simulink model "program_nova_torque_vectoring_001_2015b"  (R2016a)
settings: Solver=FixedStepAuto  StartTime=0.0  StopTime=10.0  RelTol=1e-3
PreLoadFcn:
  | dataCar
  | load_vars
  | readFuzzyFile
  | structAero
  | structEstimPar
  | structSensors
  | structSettings
PostLoadFcn:
  | , if any(exist('dsrtsu_mdlpostloadfcn', 'file') == [2, 3, 6]), try dsrtsu_mdlpostloadfcn('Execute', bdroot); catch fprintf('Error in PostLoadFcn (dsrtsu_mdlpostloadfcn) for model "%s":\n %s\n', bdroot, lasterr); end, end,
InitFcn:
  | dataCar
  | load_vars
  | readFuzzyFile
  | structAero
  | structEstimPar
  | structSensors
  | structSettings
StartFcn:
  | dataCar
  | load_vars
  | readFuzzyFile
  | structAero
  | structEstimPar
  | structSensors
  | structSettings
values from neighbouring files (symbols this model uses):
  Throttle2_offset = 500    [load_vars.m]
  Throttle_limits = [0.15, 0.90, 0.16, 0.92]    [load_vars.m]
libraries: rtican x42, hdlsllib x32, simulink x3, fuzblock x1
(part 10 of 11)

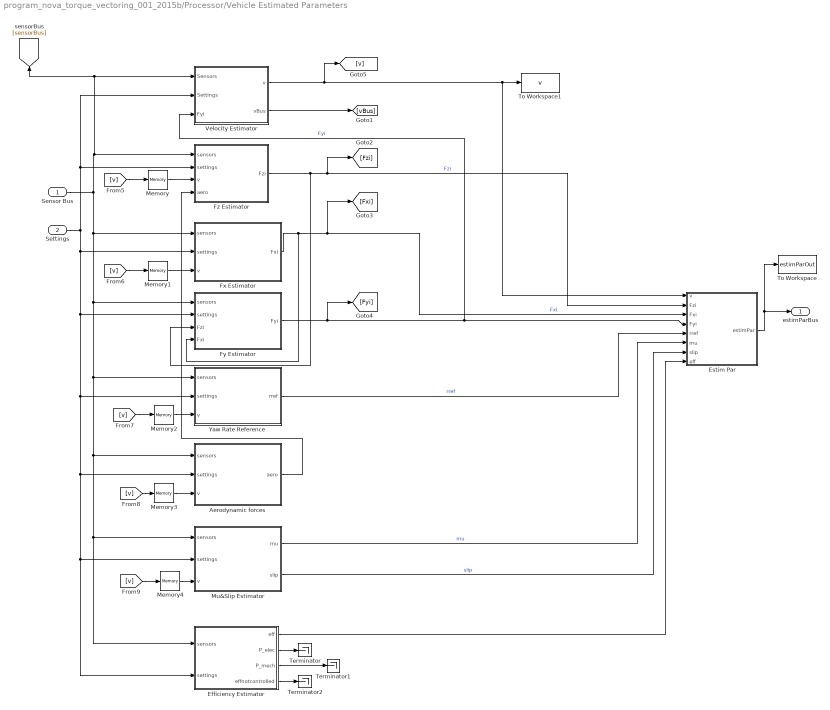
== system program_nova_torque_vectoring_001_2015b/Processor/Vehicle Estimated Parameters ==
  Sensor Bus : Inport
  Settings : Inport  Port=2
  Aerodynamic forces : MATLAB Function  TreatAsAtomicUnit=on
  Efficiency Estimator : MATLAB Function  TreatAsAtomicUnit=on
  Estim Par : MATLAB Function  TreatAsAtomicUnit=on
  "Fx Estimator " : MATLAB Function  TreatAsAtomicUnit=on
  "Fy Estimator " : MATLAB Function  TreatAsAtomicUnit=on
  "Fz Estimator " : MATLAB Function  TreatAsAtomicUnit=on
  Memory{,1..4} (5 alike) : Memory
  Mu&Slip Estimator : MATLAB Function  TreatAsAtomicUnit=on
  Terminator : Terminator
  Terminator1 : Terminator
  Terminator2 : Terminator
  To Workspace : ToWorkspace  VariableName=estimParOut  SaveFormat=Timeseries  SampleTime=-1
  To Workspace1 : ToWorkspace  VariableName=v  SaveFormat=Timeseries  SampleTime=-1
  Velocity Estimator : Subsystem
  Yaw Rate Reference : MATLAB Function  TreatAsAtomicUnit=on
  " estimParBus" : Outport
  wires:
  "Fx Estimator "/1(Fxi) -> Estim Par/3(Fxi), [Fxi], "Fy Estimator "/4(Fxi)  "Fxi"
  "Fz Estimator "/1(Fzi) -> "Fy Estimator "/3(Fzi), Estim Par/2(Fzi), [Fzi]  "Fzi"
  Yaw Rate Reference/1(rref) -> Estim Par/5(rref)  "rref"
  "Fy Estimator "/1(Fyi) -> Velocity Estimator/3(Fyi), Estim Par/4(Fyi), [Fyi]  "Fyi"
  Estim Par/1(estimPar) -> To Workspace/1, " estimParBus"/1
  Sensor Bus/1 -> "Fx Estimator "/1(sensors), Efficiency Estimator/1(sensors), Mu&Slip Estimator/1(sensors), Aerodynamic forces/1(sensors), Yaw Rate Reference/1(sensors), "Fy Estimator "/1(sensors), "Fz Estimator "/1(sensors), Velocity Estimator/1(Sensors), [sensorBus]
  Settings/1 -> Velocity Estimator/2(Settings), "Fz Estimator "/2(settings), Efficiency Estimator/2(settings), Mu&Slip Estimator/2(settings), Aerodynamic forces/2(settings), Yaw Rate Reference/2(settings), "Fy Estimator "/2(settings), "Fx Estimator "/2(settings)
  Velocity Estimator/1(v) -> [v], To Workspace1/1, Estim Par/1(v)
  Velocity Estimator/2(vBus) -> [vBus]
  Aerodynamic forces/1(aero) -> "Fz Estimator "/4(aero)
  Mu&Slip Estimator/1(mu) -> Estim Par/6(mu)  "mu"
  Mu&Slip Estimator/2(slip) -> Estim Par/7(slip)  "slip"
  [v] -> Memory/1
  [v] -> Memory1/1
  [v] -> Memory2/1
  [v] -> Memory3/1
  [v] -> Memory4/1
  Memory/1 -> "Fz Estimator "/3(v)
  Memory1/1 -> "Fx Estimator "/3(v)
  Memory2/1 -> Yaw Rate Reference/3(v)
  Memory3/1 -> Aerodynamic forces/3(v)
  Memory4/1 -> Mu&Slip Estimator/3(v)
  Efficiency Estimator/1(eff) -> Estim Par/8(eff)
  Efficiency Estimator/4(effnotcontrolled) -> Terminator2/1
  Efficiency Estimator/2(P_elec) -> Terminator/1
  Efficiency Estimator/3(P_mech) -> Terminator1/1

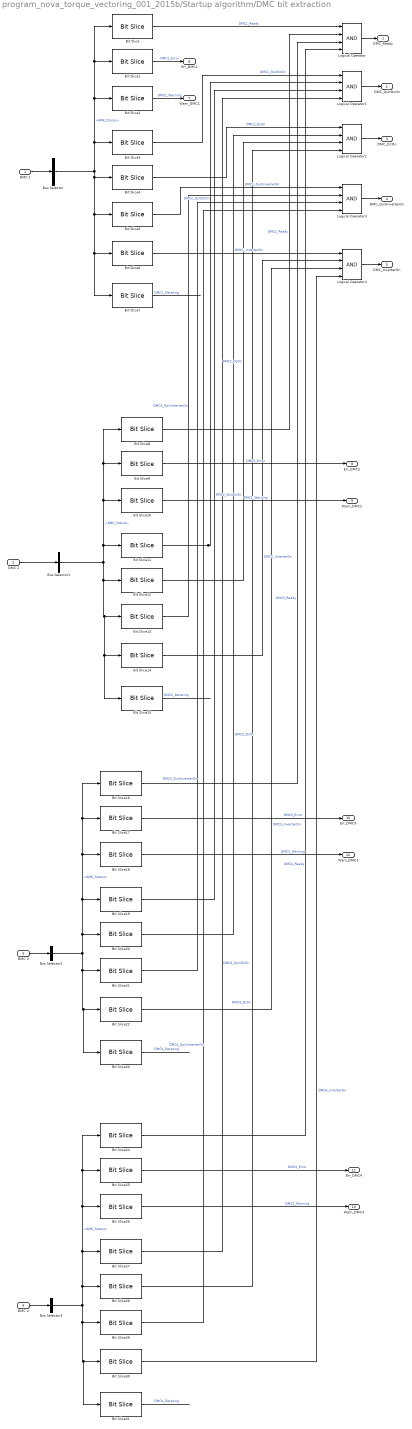
== system program_nova_torque_vectoring_001_2015b/Startup algorithm/DMC bit extraction ==
  DMC 1 : Inport
  DMC 2 : Inport  Port=2
  DMC 3 : Inport  Port=3
  DMC 4 : Inport  Port=4
  Bit Slice{,8,16,24} (4 alike) : hdlsllib/HDL Operations/Bit Slice  lidx=8  ridx=8
  Bit Slice{1,9,17,25} (4 alike) : hdlsllib/HDL Operations/Bit Slice  lidx=9  ridx=9
  Bit Slice{2,10,18,26} (4 alike) : hdlsllib/HDL Operations/Bit Slice  lidx=10  ridx=10
  Bit Slice{3,11,19,27} (4 alike) : hdlsllib/HDL Operations/Bit Slice  lidx=11  ridx=11
  Bit Slice{4,12,20,28} (4 alike) : hdlsllib/HDL Operations/Bit Slice  lidx=12  ridx=12
  Bit Slice{5,13,21,29} (4 alike) : hdlsllib/HDL Operations/Bit Slice  lidx=13  ridx=13
  Bit Slice{6,14,22,30} (4 alike) : hdlsllib/HDL Operations/Bit Slice  lidx=14  ridx=14
  Bit Slice{7,15,23,31} (4 alike) : hdlsllib/HDL Operations/Bit Slice  lidx=15  ridx=15
  Bus Selector{,1..3} (4 alike) : BusSelector  OutputSignals=AMK_Status
  Logical Operator{,1..4} (5 alike) : Logic  Inputs=4  AllPortsSameDT=off  OutDataTypeStr=boolean
  DMC_Ready : Outport
  DMC_QuitDcOn : Outport  Port=2
  DMC_DcOn : Outport  Port=3
  DMC_QuitInverterOn : Outport  Port=4
  DMC_InverterOn : Outport  Port=5
  Err_DMC1 : Outport  Port=6
  Warn_DMC1 : Outport  Port=7
  Err_DMC2 : Outport  Port=8
  Warn_DMC2 : Outport  Port=9
  Err_DMC3 : Outport  Port=10
  Err_DMC4 : Outport  Port=11
  Warn_DMC3 : Outport  Port=12
  Warn_DMC4 : Outport  Port=13
  wires:
  DMC 4/1 -> Bus Selector3/1
  DMC 3/1 -> Bus Selector2/1
  DMC 1/1 -> Bus Selector/1
  DMC 2/1 -> Bus Selector1/1
  Bus Selector/1 -> Bit Slice7/1, Bit Slice6/1, Bit Slice5/1, Bit Slice4/1, Bit Slice/1, Bit Slice1/1, Bit Slice2/1, Bit Slice3/1  "<AMK_Status>"
  Bit Slice/1 -> Logical Operator/1  "DMC1_Ready"
  Bit Slice1/1 -> Err_DMC1/1  "DMC1_Error"
  Bit Slice2/1 -> Warn_DMC1/1  "DMC1_Warning"
  Bit Slice3/1 -> Logical Operator1/1  "DMC1_QuitDcOn"
  Bit Slice4/1 -> Logical Operator2/1  "DMC1_DcOn"
  Bit Slice5/1 -> Logical Operator3/1  "DMC1_QuitInverterOn"
  Bit Slice6/1 -> Logical Operator4/1  "DMC1_InverterOn"
  Bit Slice7/1 -> ?  "DMC1_Derating"
  Bus Selector1/1 -> Bit Slice15/1, Bit Slice14/1, Bit Slice13/1, Bit Slice12/1, Bit Slice8/1, Bit Slice9/1, Bit Slice10/1, Bit Slice11/1  "<AMK_Status>"
  Bit Slice8/1 -> Logical Operator/2  "DMC2_Ready"
  Bit Slice9/1 -> Err_DMC2/1  "DMC2_Error"
  Bit Slice10/1 -> Warn_DMC2/1  "DMC2_Warning"
  Bit Slice11/1 -> Logical Operator1/2  "DMC2_QuitDcOn"
  Bit Slice12/1 -> Logical Operator2/3  "DMC2_DcOn"
  Bit Slice13/1 -> Logical Operator3/2  "DMC2_QuitInverterOn"
  Bit Slice14/1 -> Logical Operator4/2  "DMC2_InverterOn"
  Bit Slice15/1 -> ?  "DMC2_Derating"
  Bus Selector2/1 -> Bit Slice16/1, Bit Slice17/1, Bit Slice18/1, Bit Slice19/1, Bit Slice20/1, Bit Slice23/1, Bit Slice22/1, Bit Slice21/1  "<AMK_Status>"
  Bit Slice16/1 -> Logical Operator/3  "DMC3_Ready"
  Bit Slice17/1 -> Err_DMC3/1  "DMC3_Error"
  Bit Slice18/1 -> Warn_DMC3/1  "DMC3_Warning"
  Bit Slice19/1 -> Logical Operator1/3  "DMC3_QuitDcOn"
  Bit Slice20/1 -> Logical Operator2/2  "DMC3_DcOn"
  Bit Slice21/1 -> Logical Operator3/3  "DMC3_QuitInverterOn"
  Bit Slice22/1 -> Logical Operator4/3  "DMC3_InverterOn"
  Bit Slice23/1 -> ?  "DMC3_Derating"
  Bus Selector3/1 -> Bit Slice24/1, Bit Slice25/1, Bit Slice26/1, Bit Slice27/1, Bit Slice28/1, Bit Slice31/1, Bit Slice30/1, Bit Slice29/1  "<AMK_Status>"
  Bit Slice24/1 -> Logical Operator/4  "DMC4_Ready"
  Bit Slice25/1 -> Err_DMC4/1  "DMC4_Error"
  Bit Slice26/1 -> Warn_DMC4/1  "DMC4_Warning"
  Bit Slice27/1 -> Logical Operator1/4  "DMC4_QuitDcOn"
  Bit Slice28/1 -> Logical Operator2/4  "DMC4_DcOn"
  Bit Slice29/1 -> Logical Operator3/4  "DMC4_QuitInverterOn"
  Bit Slice30/1 -> Logical Operator4/4  "DMC4_InverterOn"
  Bit Slice31/1 -> ?  "DMC4_Derating"
  Logical Operator/1 -> DMC_Ready/1
  Logical Operator1/1 -> DMC_QuitDcOn/1
  Logical Operator2/1 -> DMC_DcOn/1
  Logical Operator3/1 -> DMC_QuitInverterOn/1
  Logical Operator4/1 -> DMC_InverterOn/1

== system program_nova_torque_vectoring_001_2015b/Startup algorithm/Merge_Controlword ==
  Control_in : Inport
  DcOn : Inport  Port=2
  Enable : Inport  Port=3
  InverterOn : Inport  Port=4
  ErrorReset : Inport  Port=5
  Bus Creator : BusCreator  Inputs=4
  If CTRL = Null : MATLAB Function  TreatAsAtomicUnit=on
  Control : Outport
  wires:
  Enable/1 -> If CTRL = Null/3(En_in)
  InverterOn/1 -> If CTRL = Null/4(Inv_in)
  DcOn/1 -> If CTRL = Null/2(Dc_in)
  Control_in/1 -> If CTRL = Null/1(Ctrl_in)
  If CTRL = Null/1(DcOn) -> Bus Creator/1
  If CTRL = Null/2(Enable) -> Bus Creator/2
  If CTRL = Null/3(InverterOn) -> Bus Creator/3
  Bus Creator/1 -> Control/1  "Controlbits"
  ErrorReset/1 -> Bus Creator/4  "ErrorReset"

== system program_nova_torque_vectoring_001_2015b/Processor/Control Systems/Distributor ==
  sensors : Inport
  settings : Inport  Port=2
  estimPar : Inport  Port=3
  Mz : Inport  Port=4
  MATLAB Function : MATLAB Function  TreatAsAtomicUnit=on
  MdesFdesFxmaxFx : Scope  NumInputPorts=4
  Mux : Mux
  To Workspace : ToWorkspace  VariableName=Fdes  SaveFormat=Timeseries  SampleTime=-1
  To Workspace1 : ToWorkspace  VariableName=Fxmax  SaveFormat=Timeseries  SampleTime=-1
  To Workspace2 : ToWorkspace  VariableName=MdesFdesFxmaxFx  SaveFormat=Timeseries  SampleTime=-1
  To Workspace4 : ToWorkspace  VariableName=Fx  SaveFormat=Timeseries  SampleTime=-1
  Torque/Brake analyzer : Subsystem
  torqueDistribution : Outport
  slipSet : Outport  Port=2
  wires:
  MATLAB Function/1(torqueDistribution) -> torqueDistribution/1
  sensors/1 -> Torque/Brake analyzer/1(sensors), MATLAB Function/1(sensors)
  settings/1 -> Torque/Brake analyzer/2(settings), MATLAB Function/2(settings)
  estimPar/1 -> Torque/Brake analyzer/3(estimPar), MATLAB Function/3(estimPar)
  Mz/1 -> Mux/1, MATLAB Function/4(Mz)
  MATLAB Function/2(slipSet) -> slipSet/1
  MATLAB Function/3(Fdes) -> Mux/2, MdesFdesFxmaxFx/1, To Workspace/1
  MATLAB Function/4(sumFx) -> MdesFdesFxmaxFx/2
  MATLAB Function/6(Fxmaxsum) -> MdesFdesFxmaxFx/4
  Mux/1 -> To Workspace2/1
  MATLAB Function/7(Fx) -> To Workspace4/1, Mux/4
  MATLAB Function/5(Fxmax) -> To Workspace1/1, MdesFdesFxmaxFx/3, Mux/3
  Torque/Brake analyzer/1(Fdes) -> MATLAB Function/5("Fdes ")

== system program_nova_torque_vectoring_001_2015b/Processor/Control Systems/Power Checker ==
  Sensors : Inport
  Settings : Inport  Port=2
  "estimPar  " : Inport  Port=3
  unchecked torque : Inport  Port=4
  Power checker : MATLAB Function  TreatAsAtomicUnit=on
  CheckedTorque : Outport
  wires:
  Sensors/1 -> Power checker/1(sensors)
  Settings/1 -> Power checker/2(settings)
  Power checker/1(CheckedTorque) -> CheckedTorque/1
  "estimPar  "/1 -> Power checker/3(estimPar)
  unchecked torque/1 -> Power checker/4(UncheckedTorque)

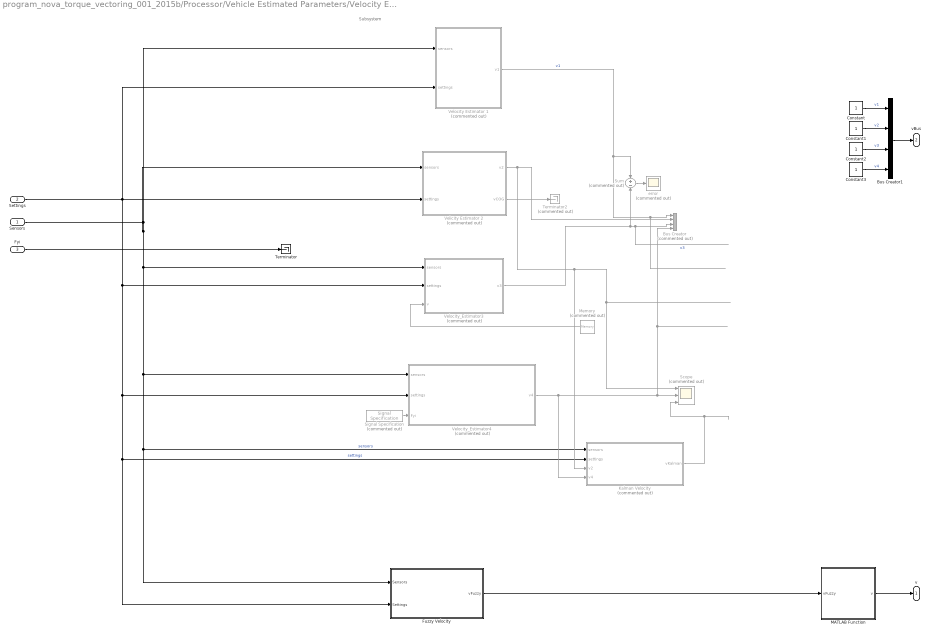
== system program_nova_torque_vectoring_001_2015b/Processor/Vehicle Estimated Parameters/Velocity Estimator ==
  note: Subsystem
  Sensors : Inport
  Settings : Inport  Port=2
  Fyi : Inport  Port=3
  Bus Creator : BusCreator  Commented=on  Inputs=4
  Bus Creator1 : BusCreator  Inputs=4
  Constant{,1..3} (4 alike) : Constant
  Fuzzy Velocity : Subsystem
  Kalman Velocity : MATLAB Function  Commented=on  TreatAsAtomicUnit=on
  MATLAB Function : MATLAB Function  TreatAsAtomicUnit=on
  Memory : Memory  Commented=on
  Scope : Scope  Commented=on  NumInputPorts=3
  Signal Specification : SignalSpecification  Commented=on  Dimensions=[4,1]
  Sum : Sum  Commented=on  Inputs=+-
  Terminator : Terminator
  Terminator2 : Terminator  Commented=on
  Velicity Estimator 2 : MATLAB Function  Commented=on  TreatAsAtomicUnit=on
  Velocity Estimator 1 : MATLAB Function  Commented=on  TreatAsAtomicUnit=on
  Velocity_Estimator3 : MATLAB Function  Commented=on  TreatAsAtomicUnit=on
  Velocity_Estimator4 : MATLAB Function  Commented=on  TreatAsAtomicUnit=on
  error : Scope  Commented=on
  v : Outport
  vBus : Outport  Port=2
  wires:
  Sensors/1 -> Velicity Estimator 2/1(sensors), Velocity_Estimator3/1(sensors), Kalman Velocity/1(sensors), Fuzzy Velocity/1(Sensors), Velocity_Estimator4/1(sensors), Velocity Estimator 1/1(sensors)  "sensors"
  Settings/1 -> Velocity_Estimator3/2(settings), Kalman Velocity/2(settings), Fuzzy Velocity/2(Settings), Velocity_Estimator4/2(settings), Velicity Estimator 2/2(settings), Velocity Estimator 1/2(settings)  "settings"
  Fuzzy Velocity/1(vFuzzy) -> MATLAB Function/1(vFuzzy)
  Velicity Estimator 2/1(v2) -> Kalman Velocity/3(v2), Scope/1, Bus Creator/2
  Velocity_Estimator4/1(v4) -> Kalman Velocity/4(v4), Bus Creator/4, Scope/2
  Kalman Velocity/1(vKalman) -> Scope/3
  MATLAB Function/1(v) -> v/1
  Signal Specification/1 -> Velocity_Estimator4/3(Fyi)
  Velocity_Estimator3/1(v3) -> Bus Creator/3, Sum/2  "v3"
  Velocity Estimator 1/1(v1) -> Sum/1, Bus Creator/1  "v1"
  Velicity Estimator 2/2(vCOG) -> Terminator2/1
  Memory/1 -> Velocity_Estimator3/3(v)
  Sum/1 -> error/1
  Bus Creator1/1 -> vBus/1
  Constant/1 -> Bus Creator1/1  "v1"
  Constant2/1 -> Bus Creator1/3  "v3"
  Constant1/1 -> Bus Creator1/2  "v2"
  Constant3/1 -> Bus Creator1/4  "v4"
  Fyi/1 -> Terminator/1

== system program_nova_torque_vectoring_001_2015b/Processor/Control Systems/Distributor/Torque//Brake analyzer ==
  sensors : Inport
  settings : Inport  Port=2
  estimPar : Inport  Port=3
  MATLAB Function1 : MATLAB Function  TreatAsAtomicUnit=on
  Fdes : Outport
  wires:
  MATLAB Function1/1(Fdes) -> Fdes/1
  sensors/1 -> MATLAB Function1/1(sensors)
  settings/1 -> MATLAB Function1/2(settings)
  estimPar/1 -> MATLAB Function1/3(estimPar)

== system program_nova_torque_vectoring_001_2015b/Processor/Vehicle Estimated Parameters/Velocity Estimator/Fuzzy Velocity ==
  Sensors : Inport
  Settings : Inport  Port=2
  Demux : Demux  Outputs=5
  FuzzyVelicityGenerator : MATLAB Function  TreatAsAtomicUnit=on
  FuzzyVelocityEstimatorConstant : fuzblock/Fuzzy Logic  Controller  fis=fuzzyVelocityEstimatorConstant
  Memory1 : Memory
  Mux : Mux  Inputs=5
  Mux1 : Mux
  To Workspace : ToWorkspace  VariableName=deltaV  SaveFormat=Timeseries  SampleTime=-1
  To Workspace1 : ToWorkspace  VariableName=maxDeltaV  SaveFormat=Timeseries  SampleTime=-1
  To Workspace2 : ToWorkspace  VariableName=ki  SaveFormat=Timeseries  SampleTime=-1
  fuzzyParam : MATLAB Function  TreatAsAtomicUnit=on
  vFuzzy : Outport
  wires:
  fuzzyParam/4(deltaVRR) -> Mux1/4, Mux/4
  fuzzyParam/2(deltaVFR) -> Mux1/2, Mux/2
  fuzzyParam/3(deltaVRL) -> Mux1/3, Mux/3
  fuzzyParam/5(maxDeltaV) -> To Workspace1/1, Mux/5
  FuzzyVelicityGenerator/1(vFuzzy) -> vFuzzy/1, Memory1/1
  fuzzyParam/1(deltaVFL) -> Mux1/1, Mux/1
  Demux/5 -> FuzzyVelicityGenerator/5(k5)
  Memory1/1 -> fuzzyParam/3(vFuzzyPrev)
  Demux/1 -> FuzzyVelicityGenerator/1(k1)
  Demux/4 -> FuzzyVelicityGenerator/4(k4)
  Demux/3 -> FuzzyVelicityGenerator/3(k3)
  Sensors/1 -> FuzzyVelicityGenerator/6(sensors), fuzzyParam/1(sensors)
  Settings/1 -> fuzzyParam/2(settings), FuzzyVelicityGenerator/7(settings)
  Demux/2 -> FuzzyVelicityGenerator/2(k2)
  Mux/1 -> FuzzyVelocityEstimatorConstant/1
  FuzzyVelocityEstimatorConstant/1 -> To Workspace2/1, Demux/1
  Mux1/1 -> To Workspace/1

== matlab function program_nova_torque_vectoring_001_2015b/Inputs/Preprocessor/MATLAB Function ==
  data: Throttle1 input; error output; Throttle2 input; limits input; throttle output
function [error,throttle]= ThrottleSensorPreprocessor(Throttle1, Throttle2, limits)
% Variables
lowerlim1 = limits(1);
upperlim1 = limits(2);
lowerlim2 = limits(3);
upperlim2 = limits(4);

% Throttle sensor 1

if Throttle1<lowerlim1
    y1=0;
elseif Throttle1>upperlim1
    y1=1;
else
    %%schalen???
end

%Throttle sensor 2

if Throttle2<lowerlim2
    y2=0;
elseif Throttle2>upperlim2
    y2=1;
else
    %%schalen???
end


% Error
if abs(Throttle1-Throttle2) > 0.10
    error = 1;
    throttle = 0;
else
    error = 0;
    throttle = (y1+y2)/2;
end

== matlab function program_nova_torque_vectoring_001_2015b/Outputs/MATLAB Function ==
  data: Torques input; torqueFL_Pos output; torqueFL_Neg output; wheelspeedFL output; torqueFR_Pos output; torqueFR_Neg output; wheelspeedFR output; torqueRL_Pos output; torqueRL_Neg output; wheelspeedRL output; torqueRR_Pos output; torqueRR_Neg output; wheelspeedRR output; status input
function [torqueFL_Pos, torqueFL_Neg, wheelspeedFL, ...
    torqueFR_Pos, torqueFR_Neg, wheelspeedFR, ...
    torqueRL_Pos, torqueRL_Neg, wheelspeedRL, ...
    torqueRR_Pos, torqueRR_Neg, wheelspeedRR]= Splitter(Torques, status)

if (status == 4)

    if Torques(1) >= 0
        torqueFL_Pos = Torques(1);
        torqueFL_Neg = 0;
        wheelspeedFL = 20000;
    else
        torqueFL_Pos = 0;
        torqueFL_Neg = Torques(1);
        wheelspeedFL = 0;
    end

    if Torques(2) >= 0
        torqueFR_Pos = Torques(2);
        torqueFR_Neg = 0;
        wheelspeedFR = 20000;
    else
        torqueFR_Pos = 0;
        torqueFR_Neg = Torques(2);
        wheelspeedFR = 0;
    end

    if Torques(3) >= 0
        torqueRL_Pos = Torques(3);
        torqueRL_Neg = 0;
        wheelspeedRL = 20000;
    else
        torqueRL_Pos = 0;
        torqueRL_Neg = Torques(3);
        wheelspeedRL = 0;
    end

    if Torques(4) >= 0
        torqueRR_Pos = Torques(4);
        torqueRR_Neg = 0;
        wheelspeedRR = 20000;
    else
        torqueRR_Pos = 0;
        torqueRR_Neg = Torques(4);
        wheelspeedRR = 0;
    end
else
    torqueFL_Pos = 0;
    torqueFL_Neg = 0;
    wheelspeedFL = 0;
    torqueFR_Pos = 0;
    torqueFR_Neg = 0;
    wheelspeedFR = 0;
    torqueRL_Pos = 0;
    torqueRL_Neg = 0;
    wheelspeedRL = 0;
    torqueRR_Pos = 0;
    torqueRR_Neg = 0;
    wheelspeedRR = 0;
end

== matlab function program_nova_torque_vectoring_001_2015b/Inputs/Preprocessor/Throttle1 perc ==
  data: u input; y output
function y = percentage(u)
%#codegen

y = u/65536;

== matlab function program_nova_torque_vectoring_001_2015b/Inputs/Preprocessor/Throttle2 perc off ==
  data: u input; y output; offset input
function y = percoff(u, offset)
%#codegen
t = u-offset
y = t/65536;

== matlab function program_nova_torque_vectoring_001_2015b/Inputs/Preprocessor/Acc conversion ==
  data: x input; y input; z input; AccX output; AccY output; AccZ output
function [AccX,AccY,AccZ] = AccConv(x,y,z)
%#codegen

AccX = x*9.81;
AccY = y*9.81;
AccZ = z*9.81;

== matlab function program_nova_torque_vectoring_001_2015b/Inputs/Preprocessor/YR//RR conversion ==
  data: y input; r input; Y output; R output
function [Y,R] = YRRR(y,r)
%#codegen

Y = y*10*2*pi;
R = r*10*2*pi;

== matlab function program_nova_torque_vectoring_001_2015b/Inputs/Preprocessor/Steering conv ==
  data: u input; Steering output
function Steering = steeringangle(u)
%#codegen

Steering = u;

== matlab function program_nova_torque_vectoring_001_2015b/Inputs/EnergyMeter/parseCurrent  ==
  data: Mux input; current output; status input; messageNr input; valueHigh input; valueLow input
function current = value(Mux,status,messageNr,valueHigh,valueLow)
%    format hex;
    valueHigh = swapbytes(typecast(valueHigh,'uint16'));
    valueLow = swapbytes(typecast(valueLow,'uint16'));
    current=0;
    %0 is current
%     disp (Mux);
%     disp (status);
%     disp (messageNr);
%     disp (valueHigh);
%     disp (valueLow);
    value = [valueHigh,valueLow];
%     disp (value);
    if Mux==0
        if status==0
            %status ok
            current = swapbytes(typecast(value,'uint32'));%current in mA
        else
        end
    end
%     disp (current);
%     format long;
%     disp (current);
end

== matlab function program_nova_torque_vectoring_001_2015b/Inputs/EnergyMeter/parseVoltage1 ==
  data: Mux input; voltage1 output; status input; messageNr input; valueHigh input; valueLow input
function voltage1 = value(Mux,status,messageNr,valueHigh,valueLow)
%    format hex;
    valueHigh = swapbytes(typecast(valueHigh,'uint16'));
    valueLow = swapbytes(typecast(valueLow,'uint16'));
    voltage1=0;
    %0 is current
%     disp (Mux);
%     disp (status);
%     disp (messageNr);
%     disp (valueHigh);
%     disp (valueLow);
    value = [valueHigh,valueLow];
%     disp (value);
    if Mux==1
        if status==0
            %status ok
            voltage1 = swapbytes(typecast(value,'uint32'));%current in mA
        else
        end
    end
%     disp (current);
%     format long;
%     disp (current);
end

== matlab function program_nova_torque_vectoring_001_2015b/Inputs/EnergyMeter/parseVoltage3 ==
  data: Mux input; voltage3 output; status input; messageNr input; valueHigh input; valueLow input
function voltage3 = value(Mux,status,messageNr,valueHigh,valueLow)
%    format hex;
    valueHigh = swapbytes(typecast(valueHigh,'uint16'));
    valueLow = swapbytes(typecast(valueLow,'uint16'));
    voltage3=0;
    %0 is current
%     disp (Mux);
%     disp (status);
%     disp (messageNr);
%     disp (valueHigh);
%     disp (valueLow);
    value = [valueHigh,valueLow];
%     disp (value);
    if Mux==3
        if status==0
            %status ok
            voltage3 = swapbytes(typecast(value,'uint32'));%current in mA
        else
        end
    end
%     disp (current);
%     format long;
%     disp (current);
end

== matlab function program_nova_torque_vectoring_001_2015b/Inputs/EnergyMeter/parseTemperature ==
  data: Mux input; temperature output; status input; messageNr input; valueHigh input; valueLow input
function temperature = value(Mux,status,messageNr,valueHigh,valueLow)
%    format hex;
    valueHigh = swapbytes(typecast(valueHigh,'uint16'));
    valueLow = swapbytes(typecast(valueLow,'uint16'));
    temperature=0;
    %0 is current
%     disp (Mux);
%     disp (status);
%     disp (messageNr);
%     disp (valueHigh);
%     disp (valueLow);
    value = [valueHigh,valueLow];
%     disp (value);
    if Mux==4
        if status==0
            %status ok
            temperature = swapbytes(typecast(value,'uint32'));%current in mA
        else
        end
    end
%     disp (current);
%     format long;
%     disp (current);
end

== matlab function program_nova_torque_vectoring_001_2015b/Inputs/EnergyMeter/parseEnergy ==
  data: Mux input; energy output; status input; messageNr input; valueHigh input; valueLow input
function energy = value(Mux,status,messageNr,valueHigh,valueLow)
%    format hex;
    valueHigh = swapbytes(typecast(valueHigh,'uint16'));
    valueLow = swapbytes(typecast(valueLow,'uint16'));
    energy=0;
    %0 is current
%     disp (Mux);
%     disp (status);
%     disp (messageNr);
%     disp (valueHigh);
%     disp (valueLow);
    value = [valueHigh,valueLow];
%     disp (value);
    if Mux==5
        if status==0
            %status ok
            energy = swapbytes(typecast(value,'uint32'));%current in mA
        else
        end
    end
%     disp (current);
%     format long;
%     disp (current);
end

== matlab function program_nova_torque_vectoring_001_2015b/Inputs/EnergyMeter/MATLAB Function ==
  data: muxByte input; response output; response0 input; response1 input; response2 input; response3 input; response4 input; response5 input; response6 input
function response = response(muxByte,response0, response1,response2,response3,response4,response5,response6)
    error = uint8(255);
    if (muxByte >= 128 && muxByte < 144)
       %error/log data
       if (muxByte < 130) % 0x82
          response = error;
       end
       if (muxByte == 130||muxByte == 131) %response on overal logdata, 0x82 en 0x83
           response = [response0, response1, response2, response3, response4, response5, response6];
       end
    end
    if (muxByte >=144 && muxByte < 160)
       %can id 
       switch muxByte
           case 144
           case 145
           case 146
           case 147
           case 148
           case 149
           case 150
           case 151
           case 157
           case 159
           otherwise
               response = error;
       end               
    end
    if (muxByte >=160 && muxByte < 176)
       %config result
       %cases zoals bij 90
       %default
       response = error;
    end
    if (muxByte >=176 && muxByte < 192)
        %set en get commands
        %B0 - B6, B9 - BC
        response = error;
    end
    if (muxByte == 255)
        response = error;
    end
end

== matlab function program_nova_torque_vectoring_001_2015b/Setup/MATLAB Function ==
  data: messageByte0 output; messageByte1 output; messageByte2 output; messageByte3 output; messageByte4 output; messageByte5 output; messageByte6 output; messageByte7 output; progress output; initialProgress input
function [messageByte0,messageByte1,messageByte2,messageByte3, messageByte4, messageByte5, messageByte6,messageByte7,progress] = setup(initialProgress)
    progress = initialProgress;
    messageValue = uint8(zeros(1,8));
    if (progress<5)
        if(progress==0)
            messageValue(1) = uint8(52); %0x34 set_mode --> stop
            messageValue(2:8)= uint8(zeros(1,7));
            progress=1;
        elseif(progress==1)
            messageValue(1) = uint8(33); %0x21 set configuration of U1
            messageValue(2) = uint8(2); %0x02 cyclisch && big endian
            messageValue(3:4) = uint8([0 50]); %50ms 
            messageValue(5:8) = zeros(1,4);
            progress=2;
        elseif(progress==2)
            messageValue(1) = uint8(37); %0x25 set configuration of W
            messageValue(2) = uint8(2); %0x02 cyclisch && big endian
            messageValue(3:4) = uint8([0 50]); %50ms 
            messageValue(5:8) = zeros(1,4);
            progress = 3;
        elseif(progress ==3)
            messageValue(1) = uint8(38); %0x26 set configuration of As
            messageValue(2) = uint8(2); %0x02 cyclisch && big endian
            messageValue(3:4) = uint8([0 50]); %50ms 
            messageValue(5:8) = zeros(1,4);
            progress = 4;
        elseif (progress ==4)
            messageValue(1) = uint8(52); %0x34 set_mode--> start
            messageValue(2:3) = uint8(ones(1,2));
            messageValue(4:8) = zeros(1,5);
            progress=5;
        end
        messageByte0 = messageValue(1);
        messageByte1 = messageValue(2);
        messageByte2 = messageValue(3);
        messageByte3 = messageValue(4);
        messageByte4 = messageValue(5);
        messageByte5 = messageValue(6);
        messageByte6 = messageValue(7);
        messageByte7 = messageValue(8);
    end
end

== matlab function program_nova_torque_vectoring_001_2015b/Processor/Lode Torque Conversion Block ==
  data: currentFL input; torqueFL output; currentFR input; currentRL input; currentRR input; torqueFR output; torqueRL output; torqueRR output
function [torqueFL,torqueFR,torqueRL,torqueRR] = torqueConversion(currentFL,currentFR,currentRL,currentRR)
ID110 = 107.2; %Converter peak current (from Ipex Pro)
%4.1837 = Nominal Current/Nominal Torque = 41A/9.8Nm (from AMK data sheet)

IqFL = currentFL * ID110 / 16384; %I_q (AMK manual P65)
torqueFL = IqFL / 4.1837; %T (AMK manual P65)

IqFR = currentFR * ID110 / 16384; %I_q (AMK manual P65)
torqueFR = IqFR / 4.1837; %T (AMK manual P65)

IqRL = currentRL * ID110 / 16384; %I_q (AMK manual P65)
torqueRL = IqRL / 4.1837; %T (AMK manual P65)

IqRR = currentRR * ID110 / 16384; %I_q (AMK manual P65)
torqueRR = IqRR / 4.1837; %T (AMK manual P65)

== matlab function program_nova_torque_vectoring_001_2015b/Inputs/EnergyMeter/parseVoltage2 ==
  data: Mux input; voltage2 output; status input; messageNr input; valueHigh input; valueLow input
function voltage2 = value(Mux,status,messageNr,valueHigh,valueLow)
%    format hex;
    valueHigh = swapbytes(typecast(valueHigh,'uint16'));
    valueLow = swapbytes(typecast(valueLow,'uint16'));
    voltage2=0;
    %0 is current
%     disp (Mux);
%     disp (status);
%     disp (messageNr);
%     disp (valueHigh);
%     disp (valueLow);
    value = [valueHigh,valueLow];
%     disp (value);
    if Mux==2
        if status==0
            %status ok
            voltage2 = swapbytes(typecast(value,'uint32'));%current in mA
        else
        end
    end
%     disp (current);
%     format long;
%     disp (current);
end

== matlab function program_nova_torque_vectoring_001_2015b/Inputs/EnergyMeter/parseAs ==
  data: Mux input; ampereSeconde output; status input; messageNr input; valueHigh input; valueLow input
function ampereSeconde = value(Mux,status,messageNr,valueHigh,valueLow)
%    format hex;
    valueHigh = swapbytes(typecast(valueHigh,'uint16'));
    valueLow = swapbytes(typecast(valueLow,'uint16'));
    ampereSeconde=6;
    %0 is current
%     disp (Mux);
%     disp (status);
%     disp (messageNr);
%     disp (valueHigh);
%     disp (valueLow);
    value = [valueHigh,valueLow];
%     disp (value);
    if Mux==3
        if status==0
            %status ok
            ampereSeconde = swapbytes(typecast(value,'uint32'));%current in mA
        else
        end
    end
%     disp (current);
%     format long;
%     disp (current);
end

== matlab function program_nova_torque_vectoring_001_2015b/Inputs/EnergyMeter/parseWh ==
  data: Mux input; wattHour output; status input; messageNr input; valueHigh input; valueLow input
function wattHour = value(Mux,status,messageNr,valueHigh,valueLow)
%    format hex;
    valueHigh = swapbytes(typecast(valueHigh,'uint16'));
    valueLow = swapbytes(typecast(valueLow,'uint16'));
    wattHour=0;
    %0 is current
%     disp (Mux);
%     disp (status);
%     disp (messageNr);
%     disp (valueHigh);
%     disp (valueLow);
    value = [valueHigh,valueLow];
%     disp (value);
    if Mux==7
        if status==0
            %status ok
            wattHour = swapbytes(typecast(value,'uint32'));%current in mA
        else
        end
    end
%     disp (current);
%     format long;
%     disp (current);
end

== stateflow chart program_nova_torque_vectoring_001_2015b/Startup algorithm/Startup ==
  state LVOn
    entry: AMK_Control = 1;
    entry: BMS_START= 1;
    entry: Status = 1;
  state SystemReady
    entry: BMS_START = 1;
    entry: Status = 1;
  state SwitchDCOn
    entry: Status = 2;
    entry: AMK_DcOn = 1;
  state PreparingToDrive
    entry: AMK_Enable = 1;
    entry: AMK_InverterOn = 1;
    entry: RTDS = 1;
    entry: Status = 3;
  state Running
    entry: Status = 4;
    entry: RTDS = 0;
  (default) -> LVOn
  Running -> LVOn : [Stop == 1]
  LVOn -> SystemReady : [AMK_Systemready == 1]
  PreparingToDrive -> LVOn [order 2] : [Stop ==1]
  SwitchDCOn -> LVOn [order 2] : [Stop == 1]
  SystemReady -> SwitchDCOn : [BMS_HV==1 && Start==1]
  SwitchDCOn -> PreparingToDrive [order 1] : [QuitDcOn==1 && DcOn==1]
  PreparingToDrive -> Running [order 1] : [InverterOn==1 && QuitInverterOn==1]
  data: AMK_Systemready input; BMS_HV input; AMK_Control output; AMK_DcOn output; AMK_Enable output; AMK_InverterOn output boolean; BMS_START output; RTDS output; Status output; QuitDcOn input; DcOn input; InverterOn input; QuitInverterOn input; Start input; Stop input

== matlab function program_nova_torque_vectoring_001_2015b/Inputs/Preprocessor/Brake 1 perc  ==
  data: u input; y output
function y = percentage(u)
%#codegen

y = u/65536;

== matlab function program_nova_torque_vectoring_001_2015b/Inputs/Preprocessor/Brake 2 perc  ==
  data: u input; y output
function y = percentage(u)
%#codegen

y = u/65536;

== matlab function program_nova_torque_vectoring_001_2015b/Startup algorithm/Merge_Controlword/If CTRL = Null ==
  data: Ctrl_in input; DcOn output; Dc_in input; En_in input; Inv_in input; Enable output; InverterOn output
function [DcOn, Enable, InverterOn] = fcn(Ctrl_in, Dc_in, En_in, Inv_in)
%#codegen

if (Ctrl_in==0)
    DcOn = false;
    Enable = false;
    InverterOn = false;
else
    DcOn = logical(Dc_in);
    Enable = logical(En_in);
    InverterOn = logical(Inv_in);
end

== matlab function program_nova_torque_vectoring_001_2015b/Processor/Bypass/Torque Vectoring Bypass ==
  data: settings input; torqueBypass output; sensors input; rpmBypass output; car parameter
function [torqueBypass,rpmBypass]= TV_Bypass(settings, sensors, car)
PmaxTyre = car.Pmax_bypass*0.25;
rad2rpm = 30/pi;


safetyFactor = 0.5;
torqueBypass = car.motor.Tmax*safetyFactor*car.gearRatio*sensors.throttle;

if sensors.throttle > 0
    rpmBypass = car.motor.rpmMax;
else
    rpmBypass = [0;0;0;0];
end

%% Power limiter
limit = PmaxTyre./max(sensors.wheelspeed,1);
torqueBypass = max(min(torqueBypass,limit),-limit);

== matlab function program_nova_torque_vectoring_001_2015b/Processor/Control Systems/Distributor/MATLAB Function ==
  data: sensors input; torqueDistribution output; settings input; estimPar input; car parameter; Mz input; slipSet output; Fdes output; sumFx output; Fxmax output; Fxmaxsum output; Fx output; Fdes input
function [torqueDistribution, slipSet,Fdes,sumFx,Fxmax,Fxmaxsum, Fx]= TorqueDistributor(sensors,settings, estimPar, car, Mz, Fdes)
%,Fdes,sumFx,Fxmax,Fxmaxsum

torqueDistribution = [0;0;0;0];
slipSet = [0;0;0;0];


sumFx=0;
Fxmax=[0;0;0;0];
Fxmaxsum=0;
Fx=[0;0;0;0];
if settings.torqueMode == 1
    
    dT =  0.25*Mz/(car.tw*0.5)*car.tireRadius;
    torqueDistribution = car.motor.Tmax*sensors.throttle;
    torqueDistribution = torqueDistribution + [-1; 1; -1; 1]*dT;
    
    for i=1:4
        if torqueDistribution(i) > 0
            slipSet(i) = car.TC.slipSetAcc;
        else
            slipSet(i) = car.TC.slipSetBrake;
        end
    end
    
    
end



%Test torque mode: only Fx, no steeringAngle

if settings.torqueMode == 2
    

    
    Fxmax = [0;0;0;0];
    %minForce = 2*car.Cd*car.AFront*0.5*car.rhoAir*estimPar.v*estimPar.v*0.25; %2* of niet? en met Cd?
    minForce = 0;
    %FyReduceFactor = 0.1;
    %Fxmax = (max((estimPar.mu .* estimPar.Fzi).^2-FyReduceFactor*estimPar.Fyi.^2,0).^0.5); %Kamm's circle
    
    
    
    Fxmax = estimPar.mu.*estimPar.Fzi;
    
    Fxmax = max(Fxmax,minForce);
    
    FxmaxMax = car.gearRatio*car.motor.Tmax/car.tireRadius; %make sure the max torque of the motor isn't surpassed
    checkFxmax = find((Fxmax > FxmaxMax)==1);
    Fxmax(checkFxmax)=FxmaxMax(checkFxmax);
    
    if settings.unlimitedFx == 1  %Surpass the tyre grip limits in case if the driver feels to restricted with this.
        Fxmax = FxmaxMax;
    end
    
    Fxmaxsum = sum(Fxmax);
    Fxmin = -Fxmax*settings.Regen;
    
    Fx = [0;0;0;0];
    
    
    Fx = Distributor(settings, car, Mz, Fdes, Fxmax, Fxmin);
    
    torqueDistribution = car.tireRadius*Fx; %torque of motor, NOT of wheels (as IPG expects this as input)
    
    for i=1:4
        if torqueDistribution(i) > 0
            slipSet(i) = car.TC.slipSetAcc;
        else
            slipSet(i) = car.TC.slipSetBrake;
        end
    end
    
    sumFx = sum(Fx);
end


end

== matlab function program_nova_torque_vectoring_001_2015b/Processor/Control Systems/Distributor/Torque//Brake analyzer/MATLAB Function1 ==
  data: sensors input; Fdes output; settings input; estimPar input; car parameter
function Fdes = Fdes(sensors, settings, estimPar, car)
    


%Fdes = 11*4* min(car.motor.Tmax)*variables.TD_percentage*sensors.throttle/car.tireRadius;
    %if sensors.throttle > 0
    %Fdes = sum(car.motor.Tmax)*variables.TD_percentage*sensors.throttle/car.tireRadius; % *4 because four motors
    %Fdes = Fdes*car.gearRatio;
    
    Fdes = sum(sensors.throttle*1.5*estimPar.mu*(car.mass*car.g + 0.5*car.rhoAir*estimPar.v*estimPar.v*car.Cl*car.AFront));
    
    if sensors.brake > 0
        Fdes = -sum(car.motor.Tmax)*sensors.brake/car.tireRadius;
        Fdes = Fdes*car.gearRatio;
    end
    %Fdes= 5000;
    
    %end
    %     Fdes = Fdes*1;
    %     Fdes = 800;
    
    %     Fdes = sensors.throttle*mean(estimPar.mu)*(car.mass*car.g + 0.5*car.rhoAir*estimPar.v*estimPar.v*car.Cl*car.AFront );
    %     Fdes = Fdes;
    

end

== matlab function program_nova_torque_vectoring_001_2015b/Processor/Control Systems/Power Checker/Power checker ==
  data: sensors input; settings input; estimPar input; UncheckedTorque input; CheckedTorque output; car parameter
function CheckedTorque = fcn(sensors,settings,estimPar, UncheckedTorque,car)

%% Power limiter according to FS rules

P_mech = sum(UncheckedTorque.*sensors.wheelspeed*car.gearRatio); %[Nm*rad/s][W]

maxMechPower = (car.Pmax - car.PC.safetyMargin)*estimPar.eff;
power2beReduced = 0;

if P_mech > maxMechPower
    power2beReduced = P_mech - maxMechPower;
end

if abs(P_mech) > 0.1
    part2beReduced = power2beReduced/P_mech;
else
    part2beReduced = 0;
end

CheckedTorque = UncheckedTorque*max(min((1 - part2beReduced),1),0);
CheckedP_mech = sum(CheckedTorque.*sensors.wheelspeed*car.gearRatio); %[Nm*rad/s][W]

== matlab function program_nova_torque_vectoring_001_2015b/Processor/Control Systems/Traction Control ==
  data: sensors input; Torques output; settings input; estimPar input; torqueDistribution input; slipSet input; car parameter; TiTi2 output; error output; rpmSet output
function [Torques, TiTi2, error, rpmSet] = Traction(sensors, settings, estimPar, torqueDistribution, slipSet, car)

error =[0 0 0 0]';
persistent errorInt; if isempty(errorInt); errorInt=[0 0 0 0]'; end
persistent errorD; if isempty(errorD); errorD=[0 0 0 0]'; end
persistent errorPrev; if isempty(errorPrev); errorPrev=[0 0 0 0]'; end

%persistent wi_prev; if isempty(wi_prev); wi_prev=[0 0 0 0]'; end
%persistent SR_expected; if isempty(SR_expected); SR_expected=zeros(4, 8); end
%persistent wvi_prev; if isempty(wvi_prev); wvi_prev=[0 0 0 0]'; end

persistent TiPrev; if isempty(TiPrev); TiPrev=[0 0 0 0]'; end

persistent errorInt2; if isempty(errorInt2); errorInt2=[0 0 0 0]'; end
persistent Ti; if isempty(Ti); Ti=[0 0 0 0]'; end
persistent Ti2; if isempty(Ti2); Ti2=[0 0 0 0]'; end

rpmSet = [20000;20000;20000;20000];

if settings.TC == 1

    slipRatioTarget = slipSet;
    dist = estimPar.Fzi/sum(estimPar.Fzi);
    
    Kp = 100*dist*10;
    Ki = 40*dist*1000;
    Kd = 0*dist/100;
    Kv = 70/100;
    Mu = car.mu;
    
    Kp2 = 20*dist/1000;
    Ki2 = 40*dist/1000;
    
    %normal non linear torque control
    error = slipRatioTarget - estimPar.slip;
    
    errorInt = errorInt + error*car.dt;
    errorInt = min(max(errorInt,-0.001*[1;1;1;1]),0.003*[1;1;1;1]);
    errorD = min(max(errorD*0.1 + 0.9*(error - errorPrev)/car.dt,-25),25);
    lambdaD = Kp.*error + Ki.*errorInt + Kd.*errorD;
    Ti = lambdaD*car.tireInertia*max(estimPar.v,0)^Kv/car.tireRadius + sign(torqueDistribution).*estimPar.Fzi*(Mu)*car.tireRadius;
    Ti = Ti / car.gearRatio;
    
    %optimum seeking
    dFds = dFdsCalculator(estimPar.Fxi,estimPar.slip);
    error2 = dFds - 0;
    errorInt2 = errorInt2 + error2*car.dt;
    errorInt2 = min(max(errorInt2,-500*[1;1;1;1]),500*[1;1;1;1]);
    lambdaD2 = Kp2.*error2 + Ki2.*errorInt2;
    Ti2 = lambdaD2*car.tireInertia*max(estimPar.v,0)^Kv/car.tireRadius + sign(torqueDistribution).*estimPar.Fzi*(car.TC_mu)*car.tireRadius;
    Ti2 = Ti2 / car.gearRatio;
    
    for i=1:4
        if abs(error(i)) < 0.05
            Ti(i) = Ti2(i);
        end
    end
    
    if estimPar.v < 1/3.6
        %Ti = [80 80 180 180]';
        errorInt = [0 0 0 0]';
    end

    if sensors.throttle < 0.1
        errorInt = [0 0 0 0]';
    end
    
    lowerBoundary = TiPrev - 100/car.gearRatio;
    upperBoundary = TiPrev + 100/car.gearRatio;

    Ti = min(max(Ti,lowerBoundary),upperBoundary);
    
    TiPrev = Ti;
    errorPrev = error;
    
    Torques = Ti;
    for i=1:4
        if torqueDistribution(i) > 0
            Torques(i) = max(min(Torques(i),torqueDistribution(i)),0); 
        else
            Torques(i) = min(max(Torques(i),torqueDistribution(i)),0);
        end
    end
    
    
else
    Torques = torqueDistribution;
end

checkTorquemax = find((Torques > car.motor.Tmax)==1); %Limit torques to max torque
Torques(checkTorquemax)=car.motor.Tmax(checkTorquemax);



%wi_prev = sensors.wheelspeed;
%wvi_prev = sensors.wheelspeedi;

TiTi2 = [Ti;Ti2];

end

function [dFds] = dFdsCalculator(Fx,slipRatio)
N = 6;

persistent slipVector, if isempty(slipVector); slipVector = zeros(N,4); end
persistent FxVector, if isempty(FxVector); FxVector = zeros(N,4); end


FxVector(1,:) = Fx;
slipVector(1,:) = slipRatio;

dFds = [0;0;0;0];

for i=1:4
    p1 = polyfit(slipVector(:,i),FxVector(:,i),1);
    p2 = polyfit(FxVector(:,i),slipVector(:,i),1);
    
    rico1 = p1(1);
    rico2 = 1/p2(1);
    
    rico = sign(min(abs(rico1),abs(rico2)))*min(abs(rico1),abs(rico2));

    dFds(i) = max(min(rico,20000),-20000);
end

% shift list one
dummy = FxVector(1:N-1,:);
FxVector = [[0,0,0,0];dummy];
dummy = slipVector(1:N-1,:);
slipVector = [[0,0,0,0];dummy];

end

== matlab function program_nova_torque_vectoring_001_2015b/Processor/Control Systems/Yaw Rate Control ==
  data: sensors input; Mz output; settings input; estimPar input; car parameter; error output; actions output; rref output
function [Mz,error,actions,rref]= yawRateControl(sensors, settings, estimPar, car)
%Function that controls the moment around the z-axis
%INPUTS:
%OUTPUT: Moment of the car around Z-axis [Nm]

Mz = 0;
Mz_temp = 0;
rref = estimPar.rref;
error = 0;


wheelAngle = (sensors.wheelAngles(1)+sensors.wheelAngles(2))/2;

%For analyzation
P_Action = 0;
I_Action = 0;
D_Action = 0;

steeringWheel_Action = 0;
yawRate_Action = 0;

persistent Mz_memory; if isempty(Mz_memory); Mz_memory = 0; end
persistent errorInt; if isempty(errorInt); errorInt = 0; end
persistent errorDev; if isempty(errorDev); errorDev = 0; end
persistent prevError; if isempty(prevError); prevError = 0; end
persistent prevWheelAngle; if isempty(prevWheelAngle); prevWheelAngle = 0; end
persistent prevRref; if isempty(prevRref); prevRref = 0; end


error = estimPar.rref - sensors.yawRate;
errorInt = errorInt + error*car.dt;
errorInt = min(max(errorInt,-car.YRC.intLimit),car.YRC.intLimit);
errorDev = (error - prevError)/car.dt;
wheelAngleDev = (wheelAngle - prevWheelAngle)/car.dt;
rrefDev = (estimPar.rref - prevRref)/car.dt;

velocityGain = min(max(1 - (estimPar.v - car.YRC.changeVelocity)*car.YRC.slope,0),1);

Mz_temp = (car.YRC.Kp*error + car.YRC.Ki*errorInt + car.YRC.Kd*errorDev...
    +car.YRC.Ks*wheelAngleDev + car.YRC.Kr*rrefDev)*velocityGain;
Mz_temp = max(min(Mz_temp,car.YRC.maxValue),-car.YRC.maxValue);
Mz_memory=Mz_memory+Mz_temp;

P_Action = car.YRC.Kp*error;
I_Action = car.YRC.Ki*errorInt;
D_Action = car.YRC.Kd*errorDev;
steeringWheel_Action = car.YRC.Ks*wheelAngle;
yawRate_Action = car.YRC.Kr*estimPar.rref;

actions = [P_Action;I_Action;D_Action;steeringWheel_Action;yawRate_Action];
prevError = error;
prevWheelAngle = wheelAngle;
prevRref = estimPar.rref;



% if settings.YRC == 2
%     error = estimPar.rref - sensors.yawRate;
%     integral = integral + error*car.dt;
%     derivative = (error - prevError)/car.dt;
%
%     Mz_temp = car.YRC.Kp*error + car.YRC.Ki*integral + car.YRC.Kd*derivative...
%         +car.YRC.Ks*wheelAngle + car.YRC.Kr*estimPar.rref;
%     Mz_temp = max(min(Mz_temp,car.YRC.maxValue),-car.YRC.maxValue);
%
%     prevError = error;
% end


%YRC enabled
if settings.YRC ==1
    Mz = Mz_memory;
    
    %YRC disabled
else
    Mz = 0;
end

if car.YRC.minV > estimPar.v
    Mz = 0; %if speed is too low, don't activate yaw rate control
    errorInt = 0;
    prevError = 0;
end

rref=estimPar.rref;

== matlab function program_nova_torque_vectoring_001_2015b/Processor/Controller Settings1 ==
  data: settings output Bus: settingBus; sensors input; torqueMode input; Fsens input; TC input; Power input; Regen input; unlimitedFx input; effEstimation input; YRC input
function settings  = settingController(sensors,torqueMode,Fsens,TC,Power,Regen,unlimitedFx,effEstimation,YRC)

%TODO in test: bypass met P_elec controle, altijd tenzij P_elec sensor niet werkt

%==============%
%   Options    %
% 1 settings.torqueMode : 0,1,2
% 2 settings.Fsens : 0-100 in steps of 5
% 3 settings.TC : 0 or 1 (on/off)
% 4 settings.Power : 0-100 in steps of 10
% 5 settings.Regen : 0-30 in steps of 5
% 6 settings.unlimitedFx : 0 of 1
% 7 settings.effEstimation : 0,1,2
% 8 settings.YRC : 0 or 1 (on/off)
%==============%

error_detection = 1;
if any(sensors.errors == error_detection)
    if any(sensors.TCRE == error_detection)
        TC = 0;
    end
    torqueMode = 0;
end

settings.Fxsens = 1;
settings.torqueMode = torqueMode;
settings.Fsens = Fsens;
settings.TC = TC;
settings.Power = Power;
settings.Regen = Regen;
settings.unlimitedFx = unlimitedFx;
settings.effEstimation = effEstimation;
settings.YRC = YRC;

== matlab function program_nova_torque_vectoring_001_2015b/Processor/Subsystem/MATLAB Function ==
  data: torqueController input; torques output; rpmController input; torqueBypass input; rpmBypass input; rpmRef output; settings input
function [torques,rpmRef]= Bypasser(torqueController,rpmController,torqueBypass,rpmBypass,settings)

torques = [0;0;0;0];
rpmRef = [0;0;0;0];

if settings.torqueMode == 0
    
    torques = settings.Power*torqueBypass;
    rpmRef = rpmBypass;
    
else
    
    torques = settings.Power*torqueController;
    rpmRef = rpmController;
    
end

== matlab function program_nova_torque_vectoring_001_2015b/Processor/Vehicle Estimated Parameters/Aerodynamic forces ==
  data: sensors input; aero output Bus: aeroBus; settings input; v input; car parameter
function aero = aerodynamics(sensors, settings, v, car)

% === from dataCar.m ===
% car.Cl = 3.84;      %[-]   %Lift coefficient
% car.Cd = 1.44;      %[-]   %Drag coefficient
% car.AFront = 1.3;   %[m^2] %Frontal area
% car.rhoAir = 1.225; %[kg/m^3] %air density

aero.FD = 0.5*car.Cd*car.AFront*car.rhoAir*v^2; %drag force, pointing rearward [N]
aero.FL = 0.5*car.Cl*car.AFront*car.rhoAir*v^2; %lift force, pointing upward [N]
aero.lever_FD = [-0.1;0.1]; %distance from the COG to the point of application of the drag [m]
aero.lever_FL = [-0.1;0.1]; %distance from the COG to the point of application of the lift [m]

== matlab function program_nova_torque_vectoring_001_2015b/Processor/Vehicle Estimated Parameters/Efficiency Estimator ==
  data: sensors input; eff output; settings input; car parameter; P_elec output; P_mech output; effnotcontrolled output
function [eff,P_elec,P_mech,effnotcontrolled]= Efficiency(sensors,settings,car)
%P_elec * eff = P_mech

persistent effTemp; if isempty(effTemp); effTemp = 0.7; end
persistent errorInt; if isempty(errorInt); errorInt = 0; end

Pmax = car.Pmax - car.PC.safetyMargin; %[W]

P_mech = sum(sensors.torque.*sensors.wheelspeed); %*car.gearRatio
P_elec = sensors.P_elec;
ratio = 0.2;

if settings.effEstimation == 1
    
    if P_elec > 1
        effCalc = P_mech/P_elec;
        effTemp = effTemp*ratio + (1-ratio)*min(max(effCalc,car.PC.minEff),car.PC.maxEff);
        
    elseif P_elec < 1
        effCalc = P_elec/min(P_mech,-1);
        effTemp = effTemp*ratio + (1-ratio)*min(max(effCalc,car.PC.minEff),car.PC.maxEff);
        
        
        %mogelijkheid tot uitbreiding: Pmax variable ifv van batterij voor tijdens
        %indurance
    end
    
end

if settings.effEstimation == 2
    
    if P_elec > Pmax*0.3 && sensors.throttle > 0 % only positive power limit
        
        error = (Pmax - P_elec)/Pmax;
        if error < 0 % P_elec > Pmax
            error = error*2;
        end
        
        errorInt = errorInt + error*car.dt;
        errorInt = max(min(errorInt,0.2),-0.2);
        
        dEff = car.PC.Kp*error + car.PC.Ki*errorInt; %more fitting variable name would be powerReductionFactor as this is not anymore an efficiency as Pelec * eff = Pmech
        %make car.PC.Kp velocity dependend?
        
        effTemp = max(min(effTemp + dEff,car.PC.maxEff),car.PC.minEff);
        
    else
        if P_elec > 5000
            eta = P_mech/P_elec;
            effTemp = effTemp*ratio+(1-ratio)*min(max(eta,car.PC.minEff),car.PC.maxEff);
        elseif P_elec < -5000
            eta = P_elec/min(P_mech,-1);
            effTemp = effTemp*ratio+(1-ratio)*min(max(eta,car.PC.minEff),car.PC.maxEff);
        end
        
    end
    
else
    effTemp = effTemp;
    
end


eff = effTemp;
effnotcontrolled = P_mech/P_elec;

== matlab function program_nova_torque_vectoring_001_2015b/Processor/Vehicle Estimated Parameters/Estim Par ==
  data: v input; estimPar output Bus: estimParBus; Fzi input; Fxi input; Fyi input; rref input; mu input; slip input; eff input
function estimPar = fcn(v,Fzi,Fxi,Fyi,rref,mu,slip,eff)

estimPar.v=v;
estimPar.Fzi=Fzi;
estimPar.Fxi=Fxi;
estimPar.Fyi=Fyi;
estimPar.rref=rref;
estimPar.mu=mu;
estimPar.slip=slip;
estimPar.eff=eff;

== matlab function program_nova_torque_vectoring_001_2015b/Processor/Vehicle Estimated Parameters/Fx Estimator  ==
  data: sensors input; Fxi output; settings input; v input; car parameter
function Fxi = Fx_Estimator(sensors, settings, v, car)
%OPM: gearratio zit al verwerkt in sensors.torque (= wheelTorque)

persistent wheelspeedPrev; if isempty(wheelspeedPrev); wheelspeedPrev = [0 ;0 ;0 ;0]; end
persistent inertia; if isempty(inertia); inertia = car.tireInertia; end
if isempty(v); v =0;end
wheelspeed = sensors.wheelspeed;
alpha = (wheelspeed - wheelspeedPrev)/car.dt;

%wheelTorque = car.gearRatio*sensors.torque -(car.motor.Inertia*car.gearRatio^2 - car.tireInertia)*alpha;
%to be used if only motor torque is known (real scenario)

%Fxi_est = (wheelTorque - alpha*inertia)/car.tireRadius;
Fxi_est = (sensors.torque - alpha*inertia)/car.tireRadius;
%Fxi_est = (sensors.torque)/car.tireRadius;

Fx_tot = sensors.ax*car.mass + 0.5*car.rhoAir*v^2*car.Cd*car.AFront;
Fxi = Fxi_est;




wheelspeedPrev=wheelspeed;
inertiaOut = inertia;
